simulink model "q_aero_thruster_model"  (R2023a)
settings: Solver=ode1  StartTime=0.0  StopTime=10  FixedStep=0.002  RelTol=1e-3  EnableMultiTasking=on
values from neighbouring files (symbols this model uses):
  Jeq = Jr + Jh + Jp    (= 1.1230375e-05)    [aero_param.m]
  kd = 1*10^(-5)    (= 1e-05)    [aero_param.m]
  km = 0.042    [aero_param.m]
  kt = 0.042    [aero_param.m]
  Rm = 8.4    [aero_param.m]
undefined symbols (not defined in the file or in its folder): Kpulse, Vadd
libraries: quarc_library x1
settings Model: SimulationMode=external  ExtModeTrigDuration=5000  Creator=pmartin  LastModifiedBy=brons
settings SolverCC: AlgebraicLoopSolver=TrustRegion  PositivePriorityOrder=on
settings DataIOCC: LimitDataPoints=on  SaveFormat=Array  ReturnWorkspaceOutputs=off
settings OptimizationCC: ExpressionDepthLimit=2147483647
settings DebuggingCC: UnderspecifiedInitializationDetection=Classic  MergeDetectMultiDrivingBlocksExec=none  SolverPrmCheckMsg=warning  FcnCallInpInsideContextMsg=warning  UnconnectedInputMsg=warning  UnconnectedOutputMsg=warning  UnconnectedLineMsg=warning  StateNameClashWarn=warning  SFUnexpectedBacktrackingDiag=warning  SFNoUnconditionalDefaultTransitionDiag=warning  SFExecutionAtInitializationDiag=none  ArithmeticOperatorsInVariantConditions=warning
settings ModelReferenceCC: EnableRefExpFcnMdlSchedulingChecks=on  PropagateSignalLabelsOutOfModel=off
settings SFSimCC: SimUseLocalCustomCode=off  CustomCodeUndefinedFunction=UseInterfaceOnly
settings RTWCC: Description=QUARC Win64 Target Using Toolchain  SystemTargetFile=quarc_win64.tlc  TemplateMakefile=quarc_default_tmf  RTWUseLocalCustomCode=off  Toolchain=QUARC win64 | nmake (64-bit Windows)  BuildConfiguration=Faster Runs  DLArmComputeVersion=19.05
settings CodeAppCC: StateflowObjectComments=on
settings STFCustomTargetCC: TargetLangStandard=C89/C90 (ANSI)  SystemTargetFile=quarc_win64.tlc
settings GRTTargetCC: TargetLangStandard=C89/C90 (ANSI)  ParMdlRefBuildCompliant=off  CompOptLevelCompliant=off  CombineOutputUpdateFcns=off  MatFileLogging=off  CPPClassGenCompliant=off  GRTInterface=on  ExtModeMexFile=quarc_comm
settings ConfigComp: CovMetricSettings=dw  CovSaveCumulativeToWorkspaceVar=on  CovSaveSingleToWorkspaceVar=on  CovExternalEMLEnable=off  CovSFcnEnable=off

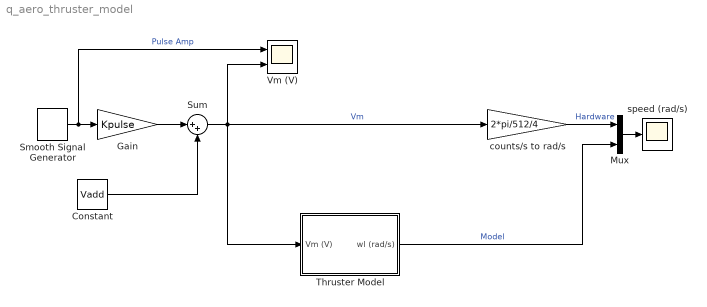
== system q_aero_thruster_model ==
  Constant : Constant  Value=Vadd
  Gain : Gain  Gain=Kpulse
  Mux : Mux  Inputs=2
  Smooth Signal Generator : quarc_library/Sources/Signals/Smooth Signal Generator  signal_type=Square  source=Internal (dialog parameters)  amplitude=1  frequency=0.5  initial_phase=0  sample_time=qc_get_step_size  output_cos=off
      settings: SourceProductName=QUARC Targets
  Sum : Sum  Inputs=|++
  Thruster Model : Subsystem
  Vm (V) : Scope  NumInputPorts=2
  counts/s to rad/s : Gain  Gain=2*pi/512/4
  speed (rad/s) : Scope
  wires:
  Thruster Model/1(wl (rad/s)) -> Mux/2  "Model"
  Smooth Signal Generator/1 -> Vm (V)/1, Gain/1  "Pulse Amp"
  Gain/1 -> Sum/1
  Constant/1 -> Sum/2
  Sum/1 -> counts/s to rad/s/1, Vm (V)/2, Thruster Model/1(Vm (V))  "Vm"
  counts/s to rad/s/1 -> Mux/1  "Hardware"
  Mux/1 -> speed (rad/s)/1

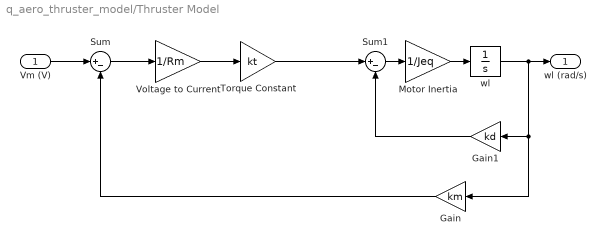
== system q_aero_thruster_model/Thruster Model ==
  Vm (V) : Inport
  Gain : Gain  Gain=km
  Gain1 : Gain  Gain=kd
  Motor Inertia : Gain  Gain=1/Jeq  SaturateOnIntegerOverflow=on  OutDataTypeStr=Inherit: Same as input  ParamDataTypeStr=Inherit: Same as input
  Sum : Sum  Inputs=|+-  InputSameDT=on  SaturateOnIntegerOverflow=on  OutDataTypeStr=Inherit: Same as first input
  Sum1 : Sum  Inputs=|+-  InputSameDT=on  SaturateOnIntegerOverflow=on  OutDataTypeStr=Inherit: Same as first input
  Torque Constant : Gain  Gain=kt
  Voltage to Current : Gain  Gain=1/Rm  SaturateOnIntegerOverflow=on  OutDataTypeStr=Inherit: Same as input  ParamDataTypeStr=Inherit: Same as input
  wl : Integrator
  wl (rad/s) : Outport
  wires:
  Voltage to Current/1 -> Torque Constant/1
  Vm (V)/1 -> Sum/1
  Sum/1 -> Voltage to Current/1
  wl/1 -> Gain/1, Gain1/1, wl (rad/s)/1
  Sum1/1 -> Motor Inertia/1
  Motor Inertia/1 -> wl/1
  Gain1/1 -> Sum1/2
  Gain/1 -> Sum/2
  Torque Constant/1 -> Sum1/1
